simulink model "poda2012B"  (R2012b)
settings: Solver=ode45  StartTime=0.0  StopTime=500  RelTol=1e-3
undefined symbols (not defined in the file): A1, A2, mi1, mi2, mu1
settings Model: Creator=Sandra Knezevic  LastModifiedBy=Aldin
settings OptimizationCC: ExpressionDepthLimit=128
settings DebuggingCC: UnderspecifiedInitializationDetection=Simplified  MergeDetectMultiDrivingBlocksExec=error  SolverPrmCheckMsg=none  FrameProcessingCompatibilityMsg=error  StateNameClashWarn=none
settings CodeAppCC: CustomSymbolStrType=$N$R$M_T
settings GRTTargetCC: CodeReplacementLibrary=C89/C90 (ANSI)

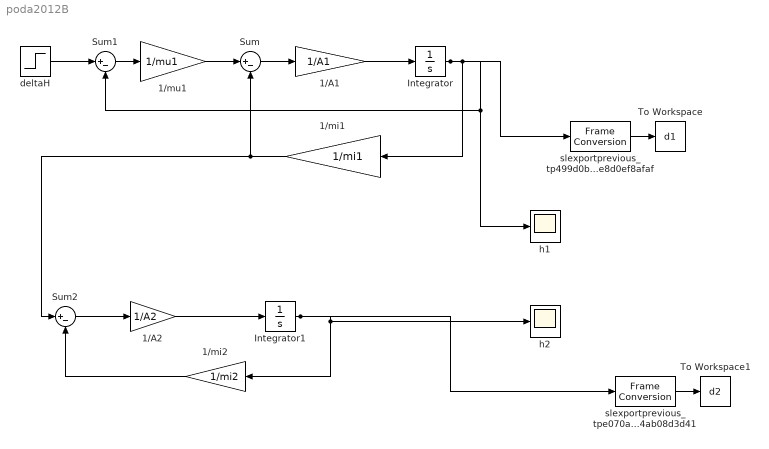
== system poda2012B ==
  1/A1 : Gain  Gain=1/A1
  1/A2 : Gain  Gain=1/A2
  1/mi1 : Gain  Gain=1/mi1
  1/mi2 : Gain  Gain=1/mi2
  1/mu1 : Gain  Gain=1/mu1
  Integrator : Integrator  InitialCondition=1
  Integrator1 : Integrator  InitialCondition=1
  Sum : Sum  Inputs=|+-
  Sum1 : Sum  Inputs=|+-
  Sum2 : Sum  Inputs=|+-
  To Workspace : ToWorkspace  VariableName=d1  SampleTime=-1
  To Workspace1 : ToWorkspace  VariableName=d2  SampleTime=-1
  deltaH : Step  After=15  SampleTime=0
  h1 : Scope
      settings: TimeRange=600  LimitDataPoints=on  MaxDataPoints=5000  SaveToWorkspace=off  SaveName=ScopeData  YMin=-10  YMax=10  SampleTime=-1  DataFormat=Array
  h2 : Scope
      settings: TimeRange=600  LimitDataPoints=on  MaxDataPoints=5000  SaveToWorkspace=off  YMin=-10  YMax=10  SampleTime=-1  DataFormat=Array
  slexportprevious_tp499d0be6_9dd3_4259_8645_6e8d0ef8afaf : FrameConversion  OutFrame=Sample-based
  slexportprevious_tpe070a98f_0d95_4aa7_a449_b64ab08d3d41 : FrameConversion  OutFrame=Sample-based
  wires:
  1/A1/1 -> Integrator/1
  1/mu1/1 -> Sum/1
  Sum/1 -> 1/A1/1
  Sum1/1 -> 1/mu1/1
  deltaH/1 -> Sum1/1
  Integrator/1 -> 1/mi1/1, Sum1/2, h1/1, slexportprevious_tp499d0be6_9dd3_4259_8645_6e8d0ef8afaf/1
  1/mi1/1 -> Sum/2, Sum2/1
  Sum2/1 -> 1/A2/1
  1/A2/1 -> Integrator1/1
  Integrator1/1 -> 1/mi2/1, h2/1, slexportprevious_tpe070a98f_0d95_4aa7_a449_b64ab08d3d41/1
  1/mi2/1 -> Sum2/2
  slexportprevious_tp499d0be6_9dd3_4259_8645_6e8d0ef8afaf/1 -> To Workspace/1
  slexportprevious_tpe070a98f_0d95_4aa7_a449_b64ab08d3d41/1 -> To Workspace1/1
